simulink model "projekatmodel"  (R2022b)
settings: Solver=VariableStepAuto  StartTime=0.0  StopTime=3000  RelTol=1e-3
libraries: fuzblock x1
settings Model: Creator=scuro  LastModifiedBy=scuro

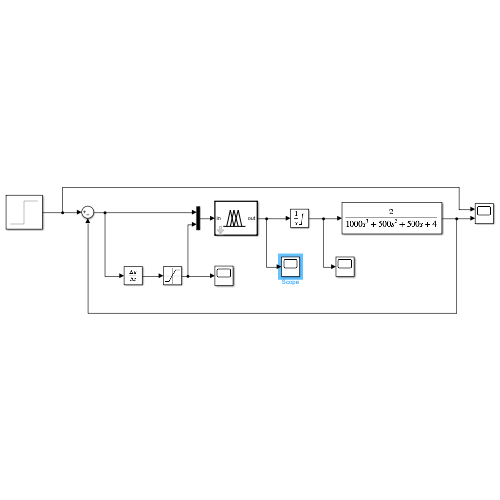
[thumbnail: Simulink's stored preview of the top-level diagram]
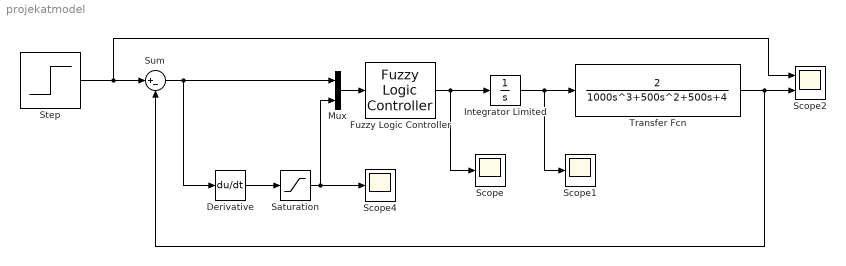
== system projekatmodel ==
  Derivative : Derivative
  Fuzzy Logic Controller : fuzblock/Fuzzy Logic  Controller  FIS='projekat.fis'  OutputSampleNumber=101  DataType=double  FuzzifiedInputs=off  RuleFiringStrengths=off  RuleOutputs=off  AggregatedOutputs=off  SimulateUsing=Interpreted execution  OutOfRangeInputValueMessage=warning  NoRuleFiredMessage=warning  EmptyOutputFuzzySetMessage=warning
  Integrator Limited : Integrator  LimitOutput=on  UpperSaturationLimit=6  LowerSaturationLimit=-6
  Mux : Mux  Inputs=2
  Saturation : Saturate  UpperLimit=1  LowerLimit=-1
  Scope : Scope
  Scope1 : Scope
  Scope2 : Scope  NumInputPorts=2
  Scope4 : Scope
  Step : Step  Time=1000  Before=-2  After=2  SampleTime=0
  Sum : Sum  Inputs=|+-
  Transfer Fcn : TransferFcn  Numerator=[2]  Denominator=[1000 500 500 4]
  wires:
  Step/1 -> Sum/1, Scope2/1
  Sum/1 -> Derivative/1, Mux/1
  Fuzzy Logic Controller/1 -> Integrator Limited/1, Scope/1
  Integrator Limited/1 -> Transfer Fcn/1, Scope1/1
  Transfer Fcn/1 -> Scope2/2, Sum/2
  Mux/1 -> Fuzzy Logic Controller/1
  Derivative/1 -> Saturation/1
  Saturation/1 -> Scope4/1, Mux/2
